simulink model "labwork2"  (R2021b)
settings: Solver=VariableStepAuto  StartTime=0.0  StopTime=10.0  RelTol=1e-3
settings Model: Creator=tshou  LastModifiedBy=Tashdid

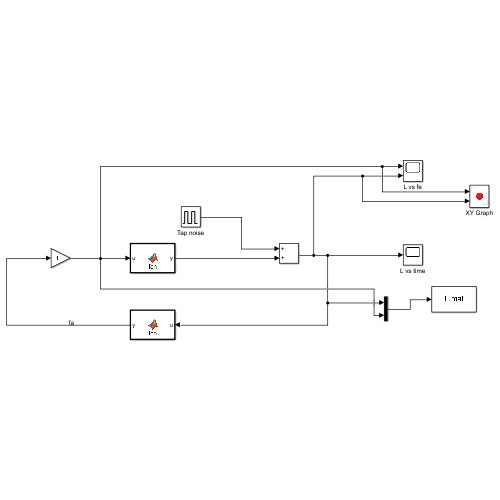
[thumbnail: Simulink's stored preview of the top-level diagram]
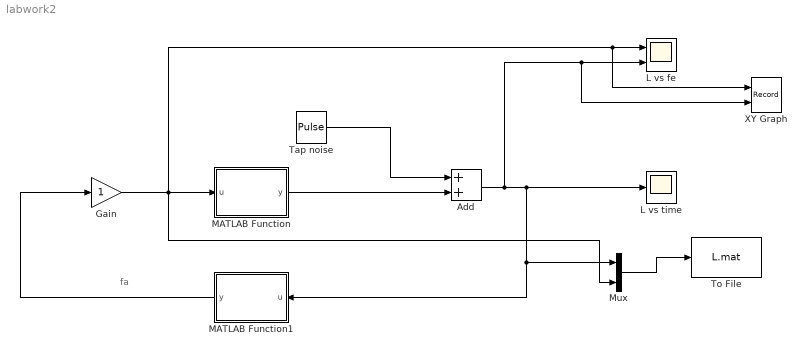
== system labwork2 ==
  note: fa
  Add : Sum
  Gain : Gain
  L vs fe : Scope  NumInputPorts=2
  L vs time : Scope
  MATLAB Function : MATLAB Function  TreatAsAtomicUnit=on
  MATLAB Function1 : MATLAB Function  TreatAsAtomicUnit=on
  Mux : Mux  Inputs=2
  Tap noise : DiscretePulseGenerator  PulseType=Time based  Period=15  PulseWidth=0.75
  To File : ToFile  Filename=L.mat
  XY Graph : Record  FileSettingsInternal="{\"entries\":[{\"content\":{\"excelSettings\":{\"content\":{},\"type\":\"Streamout.ExcelSettings\"}},\"type\":\"Streamout.FileSettingStorage\",\"uuid\":\"14199ad1-965c-486a-b58c-6f0cec685762\"}],\"packageUris\":[\"http://schema.mathworks.com/mf0/streamout_blocks/R2020a\"],\"version\":\"1.0\"}"  Layout=[1 1]  SignalsInternal="{\"entries\":[{\"content\":{\"signals\":[{\"content\":{\"blockPath\":[\"labwork2/XY Graph\"],\"channel\":[],\"dimensions\":[1],\"domain\":\"labwork2/XY Graph\",\"lineColor\":\"#a2142f\",\"plots\":[1],\"port\":1,\"sid\":[\"\"],\"signalID\":474,\"signalName\":\"Gain\"},\"type\":\"RecordBlkView.Signal\",\"uuid\":\"1943d04f-7d91-42fb-9b09-7287ca36b8f1\"},{\"content\":{\"blockPath\":[\"labwork2/XY Graph\"],\"channel\":[],\"dimensions\":[1],\"domain\":\"labwork2/XY Graph\",\"lineColor\":\"#139fff\",\"plots\":[1],\"port\":2,\"sid\":[\"\"],\"signalID\":478,\"signalName\":\"Add\"},\"type\":\"RecordBlkView.Signal\",\"uuid\":\"016fa50f-15af-41ba-ae1f-b1e9f1ade043\"}]},\"type\":\"RecordBlkView.InputSignals\",\"uuid\":\"467abf95-d1c6-4642-9dd4-1cceb2890b60\"}],\"packageUris\":[\"http://schema.mathworks.com/mf0/streamout_blocks/R2020a\"],\"version\":\"1.0\"}"  VisualizationBindings="{\"xyplotplugin\":{\"info\":[{\"series\":[{\"bindingParametersList\":[{\"parameter\":\"X-Axis\",\"signalID\":474,\"signalName\":\"Gain\"},{\"parameter\":\"Y-Axis\",\"signalID\":478,\"signalName\":\"Add\"}],\"seriesID\":1938}],\"subplotID\":1}]}}"  CompatibilityTag=XY  st=-1
  wires:
  Gain/1 -> Mux/2, XY Graph/1, L vs fe/1, MATLAB Function/1(u)
  MATLAB Function/1(y) -> Add/2
  Add/1 -> Mux/1, MATLAB Function1/1(u), L vs time/1, XY Graph/2, L vs fe/2
  MATLAB Function1/1(y) -> Gain/1
  Tap noise/1 -> Add/1
  Mux/1 -> To File/1

== matlab function labwork2/MATLAB Function ==
  data: u input; y output
function y = fcn(u)

y = 1-u^5/(0.5^5+u^5);

== matlab function labwork2/MATLAB Function1 ==
  data: u input; y output
function y = fcn(u)

y= 0.6*u*exp(0.5*u)
